simulink model "ModelWodyKaskadowej"  (R2019b)
settings: Solver=VariableStepAuto  StartTime=0.0  StopTime=10.0  RelTol=1e-3
undefined symbols (not defined in the file): A1, A2, Aw1, Aw2, fwe1, g, h10, h20
settings Model: Creator=jakub  LastModifiedBy=jakub

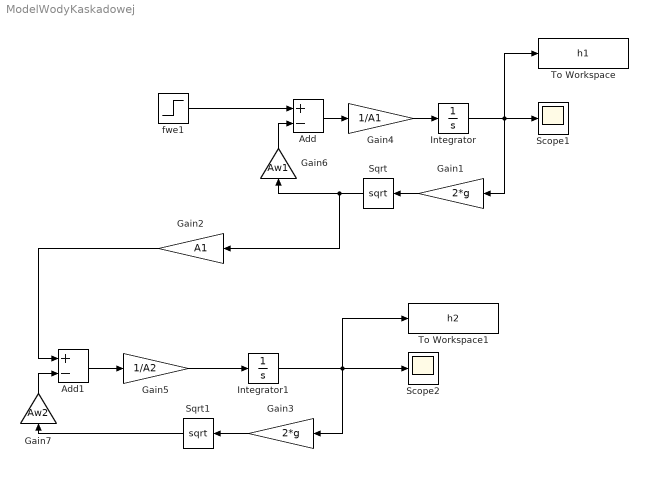
== system ModelWodyKaskadowej ==
  Add : Sum  Inputs=+-
  Add1 : Sum  Inputs=+-
  Gain1 : Gain  Gain=2*g
  Gain2 : Gain  Gain=A1
  Gain3 : Gain  Gain=2*g
  Gain4 : Gain  Gain=1/A1
  Gain5 : Gain  Gain=1/A2
  Gain6 : Gain  Gain=Aw1
  Gain7 : Gain  Gain=Aw2
  Integrator : Integrator  InitialCondition=h10
  Integrator1 : Integrator  InitialCondition=h20
  Scope1 : Scope
  Scope2 : Scope
  Sqrt : Sqrt  SaturateOnIntegerOverflow=on
  Sqrt1 : Sqrt  SaturateOnIntegerOverflow=on
  To Workspace : ToWorkspace  VariableName=h1  SampleTime=-1
  To Workspace1 : ToWorkspace  VariableName=h2  SampleTime=-1
  "fwe1 " : Step  After=fwe1  SampleTime=0
  wires:
  "fwe1 "/1 -> Add/1
  Gain1/1 -> Sqrt/1
  Add/1 -> Gain4/1
  Integrator/1 -> To Workspace/1, Scope1/1, Gain1/1
  Sqrt/1 -> Gain2/1, Gain6/1
  Add1/1 -> Gain5/1
  Integrator1/1 -> To Workspace1/1, Scope2/1, Gain3/1
  Gain3/1 -> Sqrt1/1
  Sqrt1/1 -> Gain7/1
  Gain4/1 -> Integrator/1
  Gain5/1 -> Integrator1/1
  Gain6/1 -> Add/2
  Gain7/1 -> Add1/2
  Gain2/1 -> Add1/1
